simulink model "mass_spring_damper_PD"  (R2022b)
settings: Solver=VariableStepAuto  StartTime=0.0  StopTime=100  RelTol=1e-3
settings Model: Creator=Moham  LastModifiedBy=Moham

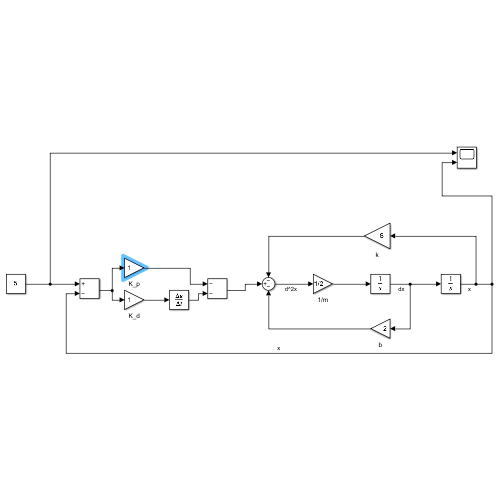
[thumbnail: Simulink's stored preview of the top-level diagram]
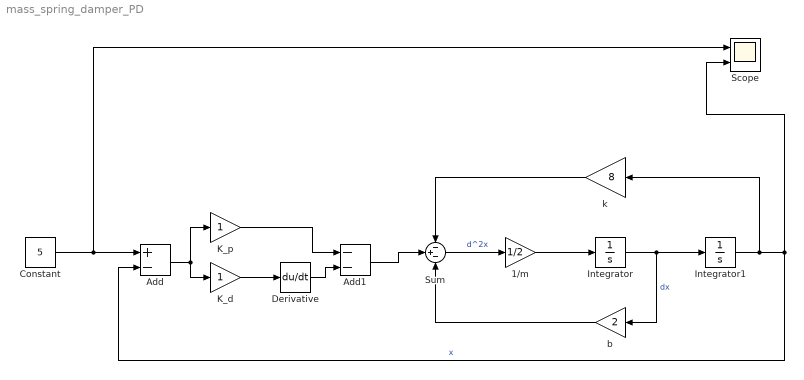
== system mass_spring_damper_PD ==
  1/m : Gain  Gain=1/2
  Add : Sum  Inputs=+-
  Add1 : Sum  Inputs=--
  Constant : Constant  Value=5
  Derivative : Derivative
  Integrator : Integrator
  Integrator1 : Integrator
  K_d : Gain
  K_p : Gain
  Scope : Scope  NumInputPorts=2
  Sum : Sum  Inputs=-+-
  b : Gain  Gain=2
  k : Gain  Gain=8
  wires:
  Integrator/1 -> b/1, Integrator1/1  "dx"
  1/m/1 -> Integrator/1
  Integrator1/1 -> Scope/2, Add/2, k/1  "x"
  Sum/1 -> 1/m/1  "d^2x"
  k/1 -> Sum/1
  b/1 -> Sum/3
  Constant/1 -> Scope/1, Add/1
  K_p/1 -> Add1/1
  K_d/1 -> Derivative/1
  Add/1 -> K_p/1, K_d/1
  Add1/1 -> Sum/2
  Derivative/1 -> Add1/2
